simulink model "otu19"  (R2018a)
settings: Solver=ode45  StartTime=0.0  StopTime=5  RelTol=1e-3  EnableMultiTasking=on
settings Model: Creator=bukova.2018  LastModifiedBy=a.pajxaev.2018
settings DataIOCC: LimitDataPoints=on  SaveFormat=Array  SignalLoggingSaveFormat=ModelDataLogs
settings OptimizationCC: ExpressionDepthLimit=2147483647  LifeSpan=inf
settings DebuggingCC: UnderspecifiedInitializationDetection=Classic  MergeDetectMultiDrivingBlocksExec=none  SolverPrmCheckMsg=warning  FcnCallInpInsideContextMsg=warning  StateNameClashWarn=warning  SFUnexpectedBacktrackingDiag=warning  SFNoUnconditionalDefaultTransitionDiag=warning  SFExecutionAtInitializationDiag=none
settings HardwareCC: ProdBitPerPointer=32  ProdBitPerSizeT=32  ProdBitPerPtrDiffT=32  ProdLargestAtomicFloat=None  ProdIntDivRoundTo=Undefined  ProdEndianess=Unspecified  ProdWordSize=32  ProdHWDeviceType=32-bit Generic
settings ModelReferenceCC: PropagateSignalLabelsOutOfModel=off
settings CodeAppCC: StateflowObjectComments=on
settings GRTTargetCC: TargetLangStandard=C89/C90 (ANSI)  GeneratePreprocessorConditionals=Disable all  CombineOutputUpdateFcns=off  GRTInterface=on
settings ConfigComp: CovMetricSettings=dw  CovHtmlReporting=on  CovSaveCumulativeToWorkspaceVar=on  CovSaveSingleToWorkspaceVar=on  CovExternalEMLEnable=off

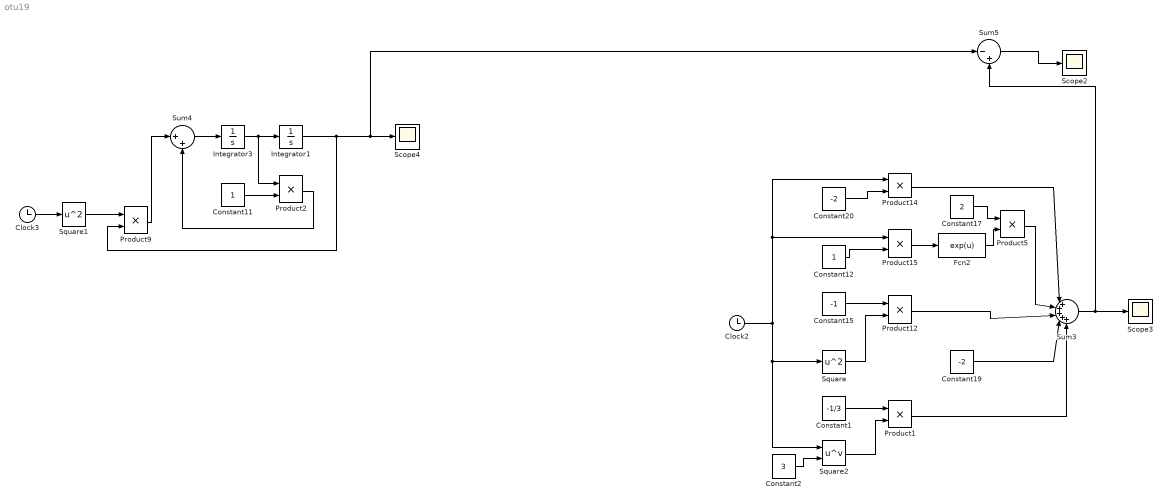
== system otu19 ==
  Clock2 : Clock
  Clock3 : Clock
  Constant1 : Constant  Value=-1/3
  Constant11 : Constant
  Constant12 : Constant
  Constant15 : Constant  Value=-1
  Constant17 : Constant  Value=2
  Constant19 : Constant  Value=-2
  Constant2 : Constant  Value=3
  Constant20 : Constant  Value=-2
  Fcn2 : Fcn  Expr=exp(u)
  Integrator1 : Integrator
  Integrator3 : Integrator
  Product{1..2,5,9,12,14..15} (7 alike) : Product  RndMeth=Zero
  Scope2 : Scope
  Scope3 : Scope
  Scope4 : Scope
  Square : Math  Operator=square  SaturateOnIntegerOverflow=on
  Square1 : Math  Operator=square  SaturateOnIntegerOverflow=on
  Square2 : Math  Operator=pow  SaturateOnIntegerOverflow=on
  Sum3 : Sum  Inputs=|+++++
  Sum4 : Sum  Inputs=|++
  Sum5 : Sum  Inputs=|-+
  wires:
  Constant19/1 -> Sum3/4
  Product5/1 -> Sum3/2
  Clock2/1 -> Product15/1, Product14/1, Square/1, Square2/1
  Constant15/1 -> Product12/1
  Product14/1 -> Sum3/1
  Product12/1 -> Sum3/3
  Constant12/1 -> Product15/2
  Clock3/1 -> Square1/1
  Integrator3/1 -> Product2/1, Integrator1/1
  Constant17/1 -> Product5/1
  Fcn2/1 -> Product5/2
  Product15/1 -> Fcn2/1
  Sum5/1 -> Scope2/1
  Constant20/1 -> Product14/2
  Sum4/1 -> Integrator3/1
  Square/1 -> Product12/2
  Sum3/1 -> Sum5/2, Scope3/1
  Product9/1 -> Sum4/1
  Square1/1 -> Product9/1
  Constant1/1 -> Product1/1
  Square2/1 -> Product1/2
  Product1/1 -> Sum3/5
  Constant2/1 -> Square2/2
  Constant11/1 -> Product2/2
  Integrator1/1 -> Product9/2, Sum5/1, Scope4/1
  Product2/1 -> Sum4/2
